simulink model "sltestAutosarTestHarnessExample"  (R2017a)
settings: Solver=FixedStepAuto  StartTime=0.0  StopTime=15  FixedStep=0.1  RelTol=1e-3  EnableMultiTasking=on
PostLoadFcn:
  | a.time = (0:0.1:15);
  | a.signals(1).values = zeros(length(a.time),1) + 10;
  | a.signals(2).values = zeros(length(a.time),1);
  | a.signals(3).values = zeros(length(a.time),1) + 15;
  | a.signals(4).values = zeros(length(a.time),1);
  | a.signals(5).values = zeros(length(a.time),1) + 20;
  | a.signals(6).values = zeros(length(a.time),1);
  | a.signals(1).dimensions = 1;
  | a.signals(2).dimensions = 1;
  | a.signals(3).dimensions = 1;
  | a.signals(4).dimensions = 1;
  | a.signals(5).dimensions = 1;
  | a.signals(6).dimensions = 1;
CloseFcn:
  | clear a;
settings Model: Creator=The MathWorks, Inc.  LastModifiedBy=The MathWorks, Inc.
settings DataIOCC: LimitDataPoints=on  SaveFormat=Array
settings OptimizationCC: DefaultParameterBehavior=Inlined  ZeroExternalMemoryAtStartup=off  ZeroInternalMemoryAtStartup=off  LifeSpan=1
settings DebuggingCC: SolverPrmCheckMsg=warning  AllowSymbolicDim=off  SFUnexpectedBacktrackingDiag=warning  SFNoUnconditionalDefaultTransitionDiag=warning  SFExecutionAtInitializationDiag=none
settings ModelReferenceCC: ModelReferenceNumInstancesAllowed=Single  PropagateSignalLabelsOutOfModel=off
settings SFSimCC: SimGenImportedTypeDefs=on  MATLABDynamicMemAlloc=off
settings RTWCC: SystemTargetFile=autosar.tlc  GenCodeOnly=on  TemplateMakefile=ert_default_tmf  Description=AUTOSAR  GenerateReport=on  IncludeHyperlinkInReport=on  LaunchReport=on  GenerateTraceInfo=on  GenerateTraceReport=on  GenerateTraceReportSl=on  GenerateTraceReportSf=on  GenerateTraceReportEml=on
settings CodeAppCC: ForceParamTrailComments=on  IgnoreCustomStorageClasses=off  OperatorAnnotations=on  SimulinkDataObjDesc=on  SFDataObjDesc=on  MATLABFcnDesc=on  InsertBlockDesc=on  MATLABSourceComments=on
settings STFCustomTargetCC: ParMdlRefBuildCompliant=on  CompOptLevelCompliant=on  IncludeMdlTerminateFcn=off  CombineOutputUpdateFcns=on  SuppressErrorStatus=on  ERTFirstTimeCompliant=on  ERTCustomFileBanners=on  SupportNonFinite=off  SupportComplex=off  SupportContinuousTime=off  SupportNonInlinedSFcns=off  RemoveResetFunc=on  MATLABClassNameForMDSCustomization=Simulink.SoftwareTarget.ERTCustomization  AutosarCompliant=on  GRTInterface=off  UseToolchainInfoCompliant=on  LookupTableObjectStructAxisOrder=2,1,3,4,...  SystemTargetFile=autosar.tlc
settings ERTTargetCC: MultiwordLength=2048  ConcurrentExecutionCompliant=off  IncludeMdlTerminateFcn=off  SuppressErrorStatus=on  SupportNonFinite=off  SupportComplex=off  ModelStepFunctionPrototypeControlCompliant=off  CPPClassGenCompliant=off  AutosarCompliant=on  LookupTableObjectStructAxisOrder=2,1,3,4,...  InlinedParameterPlacement=NonHierarchical  ERTCustomFileTemplate=example_file_process.tlc
settings ConfigComp: CovMetricSettings=dw  CovHtmlReporting=on  CovSaveCumulativeToWorkspaceVar=on  CovSaveSingleToWorkspaceVar=on  CovExternalEMLEnable=off  CovSFcnEnable=off

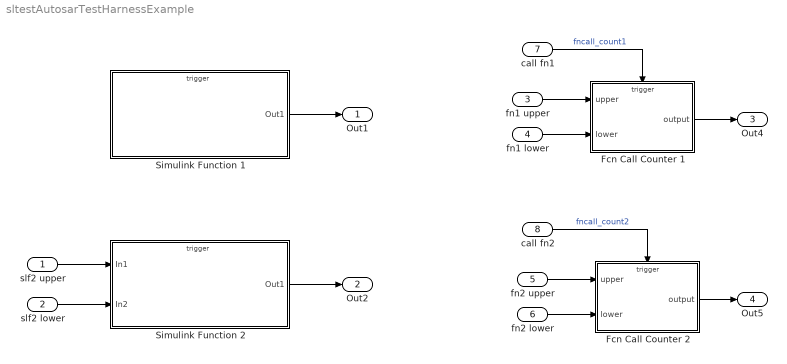
== system sltestAutosarTestHarnessExample ==
  slf2 upper : Inport
  slf2 lower : Inport  Port=2
  fn1 upper : Inport  Port=3
  fn1 lower : Inport  Port=4
  fn2 upper : Inport  Port=5
  fn2 lower : Inport  Port=6
  call fn1 : Inport  Port=7  OutputFunctionCall=on
  call fn2 : Inport  Port=8  OutputFunctionCall=on
  Fcn Call Counter 1 : Subsystem
  Fcn Call Counter 2 : Subsystem
  Simulink Function 1 : Subsystem  TreatAsAtomicUnit=on
  Simulink Function 2 : Subsystem  TreatAsAtomicUnit=on
  Out1 : Outport
  Out2 : Outport  Port=2
  Out4 : Outport  Port=3
  Out5 : Outport  Port=4
  wires:
  slf2 upper/1 -> Simulink Function 2/1(In1)
  Simulink Function 1/1(Out1) -> Out1/1
  Fcn Call Counter 1/1(output) -> Out4/1
  call fn1/1 -> Fcn Call Counter 1/Trigger  "fncall_count1"
  Fcn Call Counter 2/1(output) -> Out5/1
  call fn2/1 -> Fcn Call Counter 2/Trigger  "fncall_count2"
  fn1 upper/1 -> Fcn Call Counter 1/1(upper)
  fn1 lower/1 -> Fcn Call Counter 1/2(lower)
  fn2 upper/1 -> Fcn Call Counter 2/1(upper)
  fn2 lower/1 -> Fcn Call Counter 2/2(lower)
  slf2 lower/1 -> Simulink Function 2/2(In2)
  Simulink Function 2/1(Out1) -> Out2/1

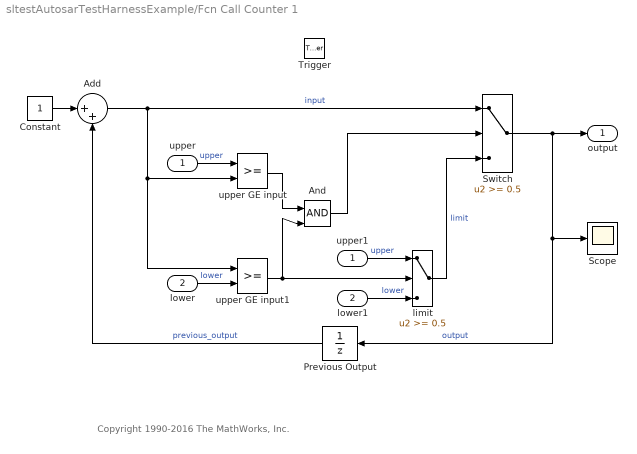
== system sltestAutosarTestHarnessExample/Fcn Call Counter 1 ==
  note: Copyright 1990-2016 The MathWorks, Inc.
  upper : Inport
  lower : Inport  Port=2
  Trigger : TriggerPort  TriggerType=function-call  VariantControl=Variant  PortDimensions=1
  " limit" : Switch  Threshold=0.5  SaturateOnIntegerOverflow=on  InputSameDT=on
  Add : Sum  Inputs=|++
  And : Logic  IconShape=distinctive  OutDataTypeStr=boolean
      settings: AttributesFormatString=%<Operator>
  Constant : Constant
  Previous Output : UnitDelay  SampleTime=-1
  Scope : Scope
  Switch : Switch  Threshold=0.5  SaturateOnIntegerOverflow=on  InputSameDT=on
  lower1 : InportShadow  Port=2
  upper GE input : RelationalOperator  Priority=0  OutDataTypeStr=boolean  RndMeth=Nearest  InputSameDT=on
      settings: AttributesFormatString=\n
  upper GE input1 : RelationalOperator  Priority=0  OutDataTypeStr=boolean  RndMeth=Nearest  InputSameDT=on
      settings: AttributesFormatString=\n
  upper1 : InportShadow
  output : Outport
  wires:
  Switch/1 -> output/1, Previous Output/1, Scope/1  "output"
  " limit"/1 -> Switch/3  "limit"
  upper GE input/1 -> And/1
  Previous Output/1 -> Add/2  "previous_output"
  upper/1 -> upper GE input/1  "upper"
  upper GE input1/1 -> And/2, " limit"/2
  And/1 -> Switch/2
  Add/1 -> Switch/1, upper GE input/2, upper GE input1/1  "input"
  Constant/1 -> Add/1
  lower/1 -> upper GE input1/2  "lower"
  upper1/1 -> " limit"/1  "upper"
  lower1/1 -> " limit"/3  "lower"

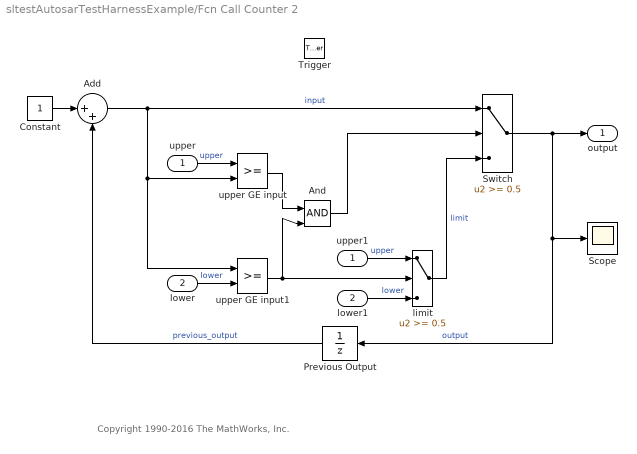
== system sltestAutosarTestHarnessExample/Fcn Call Counter 2 ==
  note: Copyright 1990-2016 The MathWorks, Inc.
  upper : Inport
  lower : Inport  Port=2
  Trigger : TriggerPort  TriggerType=function-call  VariantControl=Variant  PortDimensions=1
  " limit" : Switch  Threshold=0.5  SaturateOnIntegerOverflow=on  InputSameDT=on
  Add : Sum  Inputs=|++
  And : Logic  IconShape=distinctive  OutDataTypeStr=boolean
      settings: AttributesFormatString=%<Operator>
  Constant : Constant
  Previous Output : UnitDelay  SampleTime=-1
  Scope : Scope
  Switch : Switch  Threshold=0.5  SaturateOnIntegerOverflow=on  InputSameDT=on
  lower1 : InportShadow  Port=2
  upper GE input : RelationalOperator  Priority=0  OutDataTypeStr=boolean  RndMeth=Nearest  InputSameDT=on
      settings: AttributesFormatString=\n
  upper GE input1 : RelationalOperator  Priority=0  OutDataTypeStr=boolean  RndMeth=Nearest  InputSameDT=on
      settings: AttributesFormatString=\n
  upper1 : InportShadow
  output : Outport
  wires:
  Switch/1 -> output/1, Previous Output/1, Scope/1  "output"
  " limit"/1 -> Switch/3  "limit"
  upper GE input/1 -> And/1
  Previous Output/1 -> Add/2  "previous_output"
  upper/1 -> upper GE input/1  "upper"
  upper GE input1/1 -> And/2, " limit"/2
  And/1 -> Switch/2
  Add/1 -> Switch/1, upper GE input/2, upper GE input1/1  "input"
  Constant/1 -> Add/1
  lower/1 -> upper GE input1/2  "lower"
  upper1/1 -> " limit"/1  "upper"
  lower1/1 -> " limit"/3  "lower"

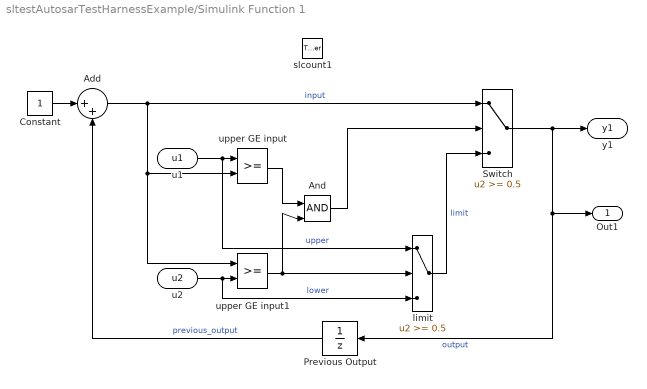
== system sltestAutosarTestHarnessExample/Simulink Function 1 ==
  slcount1 : TriggerPort  TriggerType=function-call  IsSimulinkFunction=on  FunctionName=slcount1  VariantControl=Variant
  " limit" : Switch  Threshold=0.5  SaturateOnIntegerOverflow=on  InputSameDT=on
  Add : Sum  Inputs=|++
  And : Logic  IconShape=distinctive  OutDataTypeStr=boolean
      settings: AttributesFormatString=%<Operator>
  Constant : Constant
  Previous Output : UnitDelay  SampleTime=-1
  Switch : Switch  Threshold=0.5  SaturateOnIntegerOverflow=on  InputSameDT=on
  upper GE input : RelationalOperator  Priority=0  OutDataTypeStr=boolean  RndMeth=Nearest  InputSameDT=on
      settings: AttributesFormatString=\n
  upper GE input1 : RelationalOperator  Priority=0  OutDataTypeStr=boolean  RndMeth=Nearest  InputSameDT=on
      settings: AttributesFormatString=\n
  u1 : ArgIn  DisableCoverage=on  ArgumentName=u1
  u2 : ArgIn  DisableCoverage=on  Port=2  ArgumentName=u2
  y1 : ArgOut  DisableCoverage=on  ArgumentName=y1
  Out1 : Outport
  wires:
  Switch/1 -> y1/1, Out1/1, Previous Output/1  "output"
  " limit"/1 -> Switch/3  "limit"
  upper GE input/1 -> And/1
  Previous Output/1 -> Add/2  "previous_output"
  upper GE input1/1 -> And/2, " limit"/2
  And/1 -> Switch/2
  Add/1 -> Switch/1, upper GE input/2, upper GE input1/1  "input"
  Constant/1 -> Add/1
  u1/1 -> " limit"/1, upper GE input/1  "upper"
  u2/1 -> " limit"/3, upper GE input1/2  "lower"

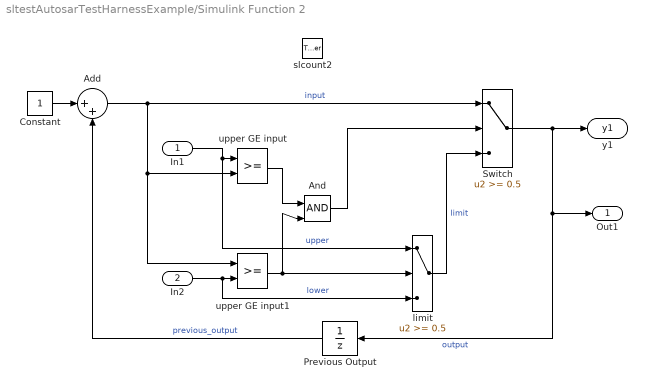
== system sltestAutosarTestHarnessExample/Simulink Function 2 ==
  In1 : Inport
  In2 : Inport  Port=2
  slcount2 : TriggerPort  TriggerType=function-call  IsSimulinkFunction=on  FunctionName=slcount2  VariantControl=Variant
  " limit" : Switch  Threshold=0.5  SaturateOnIntegerOverflow=on  InputSameDT=on
  Add : Sum  Inputs=|++
  And : Logic  IconShape=distinctive  OutDataTypeStr=boolean
      settings: AttributesFormatString=%<Operator>
  Constant : Constant
  Previous Output : UnitDelay  SampleTime=-1
  Switch : Switch  Threshold=0.5  SaturateOnIntegerOverflow=on  InputSameDT=on
  upper GE input : RelationalOperator  Priority=0  OutDataTypeStr=boolean  RndMeth=Nearest  InputSameDT=on
      settings: AttributesFormatString=\n
  upper GE input1 : RelationalOperator  Priority=0  OutDataTypeStr=boolean  RndMeth=Nearest  InputSameDT=on
      settings: AttributesFormatString=\n
  y1 : ArgOut  DisableCoverage=on  ArgumentName=y1
  Out1 : Outport
  wires:
  Switch/1 -> y1/1, Out1/1, Previous Output/1  "output"
  " limit"/1 -> Switch/3  "limit"
  upper GE input/1 -> And/1
  Previous Output/1 -> Add/2  "previous_output"
  upper GE input1/1 -> And/2, " limit"/2
  And/1 -> Switch/2
  Add/1 -> Switch/1, upper GE input/2, upper GE input1/1  "input"
  Constant/1 -> Add/1
  In1/1 -> " limit"/1, upper GE input/1  "upper"
  In2/1 -> " limit"/3, upper GE input1/2  "lower"
